simulink model "groundContactTestHarness"  (R2024a)
settings: configuration reference "standardSILConfiguraitonParams" (kept outside this file)
settings Model: Creator=jerem  LastModifiedBy=jerem
settings ConfigSetRef: SourceName=standardSILConfiguraitonParams  SourceLocation=Base Workspace

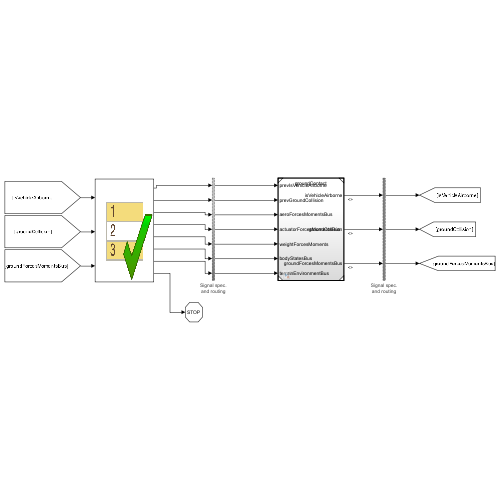
[thumbnail: Simulink's stored preview of the top-level diagram]
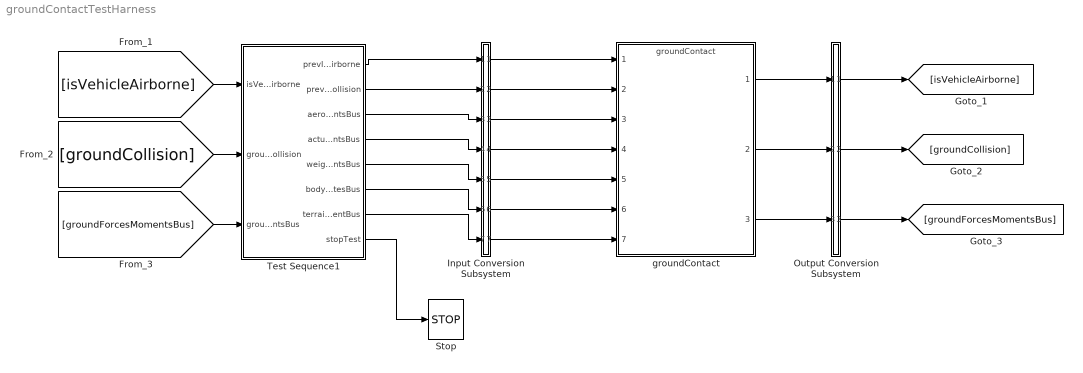
== system groundContactTestHarness ==
  Input Conversion Subsystem : Subsystem  Tag=__SLT_ICS__  Description=|
      | Signal spec.
      | and routing
      settings: AttributesFormatString=%<Description>
  Output Conversion Subsystem : Subsystem  Tag=__SLT_OCS__  Description=|
      | Signal spec.
      | and routing
      mask init:
      | ICDictionary = get_param(bdroot, 'DataDictionary');
      | if isempty(ICDictionary)
      |    ICScope = Simulink.data.BaseWorkspace;
      | else
      |    ICScope = Simulink.data.DataDictionary(ICDictionary);
      | end
      | 
      | IC3 = Simulink.Bus.createMATLABStruct('ComponentForcesMomentsBus', [], [1 1], ICScope);
      settings: AttributesFormatString=%<Description>
  Stop : Stop
  Test Sequence1 : Test Sequence  TreatAsAtomicUnit=on
  groundContact : ModelReference  ModelNameDialog=groundContact  SimulationMode=Normal  ModelReferenceVersion=1.95
  wires:
  Test Sequence1/1(prevIsVehicleAirborne) -> Input Conversion Subsystem/1(Inport_1)
  Test Sequence1/2(prevGroundCollision) -> Input Conversion Subsystem/2(Inport_2)
  Test Sequence1/3(aeroForcesMomentsBus) -> Input Conversion Subsystem/3(Inport_3)
  Test Sequence1/4(actuatorForcesMomentsBus) -> Input Conversion Subsystem/4(Inport_4)
  Test Sequence1/5(weightForcesMomentsBus) -> Input Conversion Subsystem/5(Inport_5)
  Test Sequence1/6(bodyStatesBus) -> Input Conversion Subsystem/6(Inport_6)
  Test Sequence1/7(terrainEnvironmentBus) -> Input Conversion Subsystem/7(Inport_7)
  [isVehicleAirborne] -> Test Sequence1/1(isVehicleAirborne)
  [groundCollision] -> Test Sequence1/2(groundCollision)
  [groundForcesMomentsBus] -> Test Sequence1/3(groundForcesMomentsBus)
  Output Conversion Subsystem/1(Outport_1) -> [isVehicleAirborne]
  Output Conversion Subsystem/2(Outport_2) -> [groundCollision]
  Output Conversion Subsystem/3(Outport_3) -> [groundForcesMomentsBus]
  Test Sequence1/8(stopTest) -> Stop/1
  groundContact/1 -> Output Conversion Subsystem/1(Inport_1)
  groundContact/2 -> Output Conversion Subsystem/2(Inport_2)
  groundContact/3 -> Output Conversion Subsystem/3(Inport_3)
  Input Conversion Subsystem/1(Outport_1) -> groundContact/1
  Input Conversion Subsystem/2(Outport_2) -> groundContact/2
  Input Conversion Subsystem/3(Outport_3) -> groundContact/3
  Input Conversion Subsystem/4(Outport_4) -> groundContact/4
  Input Conversion Subsystem/5(Outport_5) -> groundContact/5
  Input Conversion Subsystem/6(Outport_6) -> groundContact/6
  Input Conversion Subsystem/7(Outport_7) -> groundContact/7

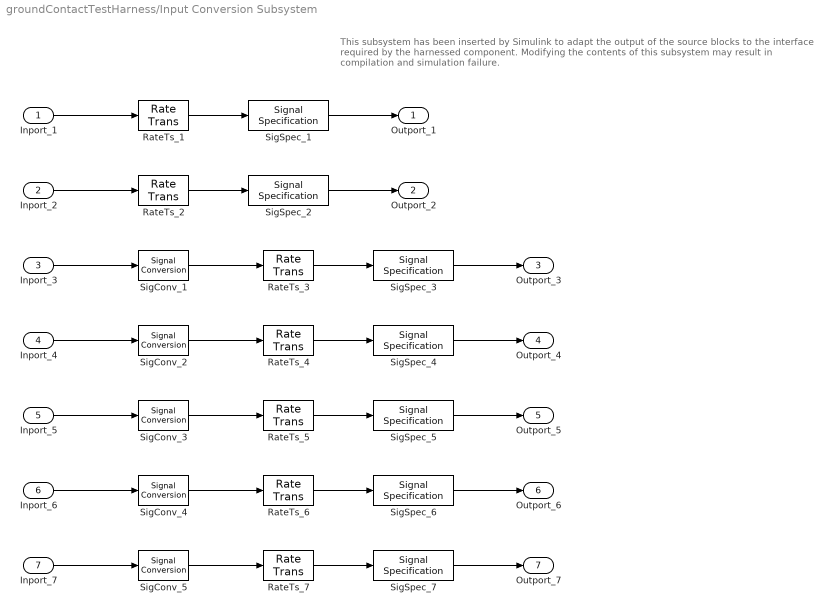
== system groundContactTestHarness/Input Conversion Subsystem ==
  note: This subsystem has been inserted by Simulink to adapt the output of the source blocks to the interface required by the harnessed component.
      |  Modifying the contents of this subsystem may result in compilation and simulation failure.
  Inport_1 : Inport
  Inport_2 : Inport  Port=2
  Inport_3 : Inport  Port=3
  Inport_4 : Inport  Port=4
  Inport_5 : Inport  Port=5
  Inport_6 : Inport  Port=6
  Inport_7 : Inport  Port=7
  RateTs_{1..7} (7 alike) : RateTransition  OutPortSampleTime=0.004
  SigConv_{1..5} (5 alike) : SignalConversion  ConversionOutput=Virtual bus  OverrideOpt=off
  SigSpec_1 : SignalSpecification  OutDataTypeStr=boolean  Dimensions=[1]  SampleTime=0.004
  SigSpec_2 : SignalSpecification  OutDataTypeStr=boolean  Dimensions=[1]  SampleTime=0.004
  SigSpec_3 : SignalSpecification  OutDataTypeStr=Bus: ComponentForcesMomentsBus  SampleTime=0.004
  SigSpec_4 : SignalSpecification  OutDataTypeStr=Bus: ComponentForcesMomentsBus  SampleTime=0.004
  SigSpec_5 : SignalSpecification  OutDataTypeStr=Bus: ComponentForcesMomentsBus  SampleTime=0.004
  SigSpec_6 : SignalSpecification  OutDataTypeStr=Bus: BodyStateBus  SampleTime=0.004
  SigSpec_7 : SignalSpecification  OutDataTypeStr=Bus: TerrainEnvironmentBus  SampleTime=0.004
  Outport_1 : Outport
  Outport_2 : Outport  Port=2
  Outport_3 : Outport  Port=3
  Outport_4 : Outport  Port=4
  Outport_5 : Outport  Port=5
  Outport_6 : Outport  Port=6
  Outport_7 : Outport  Port=7
  wires:
  SigSpec_1/1 -> Outport_1/1
  RateTs_1/1 -> SigSpec_1/1
  Inport_1/1 -> RateTs_1/1
  SigSpec_2/1 -> Outport_2/1
  RateTs_2/1 -> SigSpec_2/1
  Inport_2/1 -> RateTs_2/1
  SigSpec_3/1 -> Outport_3/1
  RateTs_3/1 -> SigSpec_3/1
  SigConv_1/1 -> RateTs_3/1
  Inport_3/1 -> SigConv_1/1
  SigSpec_4/1 -> Outport_4/1
  RateTs_4/1 -> SigSpec_4/1
  SigConv_2/1 -> RateTs_4/1
  Inport_4/1 -> SigConv_2/1
  SigSpec_5/1 -> Outport_5/1
  RateTs_5/1 -> SigSpec_5/1
  SigConv_3/1 -> RateTs_5/1
  Inport_5/1 -> SigConv_3/1
  SigSpec_6/1 -> Outport_6/1
  RateTs_6/1 -> SigSpec_6/1
  SigConv_4/1 -> RateTs_6/1
  Inport_6/1 -> SigConv_4/1
  SigSpec_7/1 -> Outport_7/1
  RateTs_7/1 -> SigSpec_7/1
  SigConv_5/1 -> RateTs_7/1
  Inport_7/1 -> SigConv_5/1

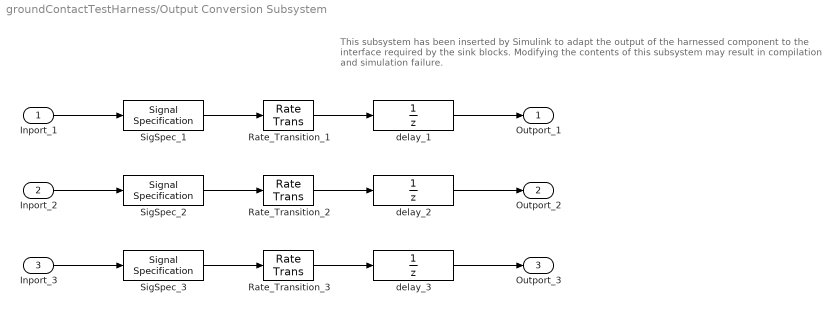
== system groundContactTestHarness/Output Conversion Subsystem ==
  note: This subsystem has been inserted by Simulink to adapt the output of the harnessed component to the interface required by the sink blocks.
      |  Modifying the contents of this subsystem may result in compilation and simulation failure.
  Inport_1 : Inport
  Inport_2 : Inport  Port=2
  Inport_3 : Inport  Port=3
  Rate_Transition_1 : RateTransition  OutPortSampleTimeOpt=Inherit
  Rate_Transition_2 : RateTransition  OutPortSampleTimeOpt=Inherit
  Rate_Transition_3 : RateTransition  OutPortSampleTimeOpt=Inherit
  SigSpec_1 : SignalSpecification  OutDataTypeStr=boolean  Dimensions=[1]  SampleTime=0.004
  SigSpec_2 : SignalSpecification  OutDataTypeStr=boolean  Dimensions=[1]  SampleTime=0.004
  SigSpec_3 : SignalSpecification  OutDataTypeStr=Bus: ComponentForcesMomentsBus  Dimensions=[1]  SampleTime=0.004
  delay_1 : UnitDelay  SampleTime=-1
  delay_2 : UnitDelay  SampleTime=-1
  delay_3 : UnitDelay  InitialCondition=IC3  SampleTime=-1
  Outport_1 : Outport
  Outport_2 : Outport  Port=2
  Outport_3 : Outport  Port=3
  wires:
  Inport_1/1 -> SigSpec_1/1
  SigSpec_1/1 -> Rate_Transition_1/1
  Rate_Transition_1/1 -> delay_1/1
  delay_1/1 -> Outport_1/1
  Inport_2/1 -> SigSpec_2/1
  SigSpec_2/1 -> Rate_Transition_2/1
  Rate_Transition_2/1 -> delay_2/1
  delay_2/1 -> Outport_2/1
  Inport_3/1 -> SigSpec_3/1
  SigSpec_3/1 -> Rate_Transition_3/1
  Rate_Transition_3/1 -> delay_3/1
  delay_3/1 -> Outport_3/1

== stateflow chart groundContactTestHarness/Test Sequence1 ==
  state Scenario_2
    state Initialize
      %% Initialize data outputs.
      stopTest = false;
      prevIsVehicleAirborne = false;
      prevGroundCollision = false;
      aeroForcesMomentsBus.forcesInBody_N = zeros(3,1);
      aeroForcesMomentsBus.momentsInBody_Nm = zeros(3,1);
      actuatorForcesMomentsBus.forcesInBody_N = zeros(3,1);
      actuatorForcesMomentsBus.momentsInBody_Nm = zeros(3,1);
      weightForcesMomentsBus.forcesInBody_N = zeros(3,1);
      weightForcesMomentsBus.momentsInBody_Nm = zeros(3,1);
      bodyStatesBus.aircraftVelInNED_mps = zeros(3,1);
      bodyStatesBus.aircraftPosInNED_m = zeros(3,1);
      bodyStatesBus.aircraftEulerAngles_rad = zeros(3,1);
      bodyStatesBus.aircraftVelInBody_mps = zeros(3,1);
      bodyStatesBus.aircraftAngVelInBody_radps = zeros(3,1);
      bodyStatesBus.aircraftAngAccelInBody_radps2 = zeros(3,1);
      bodyStatesBus.aircraftAccelInBody_mps2 = zeros(3,1);
      bodyStatesBus.DCM_be = eye(3,3);
      terrainEnvironmentBus.terrainHeightInNED_m = 0;
    state verifyInitialization
      verify(isVehicleAirborne == 0)
      verify(groundCollision == 0)
      verify(isClose(groundForcesMomentsBus.forcesInBody_N(1),0))
      verify(isClose(groundForcesMomentsBus.forcesInBody_N(2),0))
      verify(isClose(groundForcesMomentsBus.forcesInBody_N(3),0))
      verify(isClose(groundForcesMomentsBus.momentsInBody_Nm(1), 0))
      verify(isClose(groundForcesMomentsBus.momentsInBody_Nm(2), 0))
      verify(isClose(groundForcesMomentsBus.momentsInBody_Nm(3), 0))
    state stationaryOnAirstrip
      bodyStatesBus.DCM_be =  eye(3,3);
      % test some forces and moments
      aeroForcesMomentsBus.forcesInBody_N = [0; 0 ; 0]; % simulating moving on runway
      aeroForcesMomentsBus.momentsInBody_Nm = [0; 0; 0]; % Cm is naturally negative
      weightForcesMomentsBus.forcesInBody_N =[0; 0; 9298.6 * 9.81]; % weight of vehicle, must be positive (toward earth)
      weightForcesMomentsBus.momentsInBody_Nm = zeros(3,1);
    state verifyStationary
      verify(isVehicleAirborne == 0)
      verify(groundCollision == 0)
      verify(isClose(groundForcesMomentsBus.forcesInBody_N(1), 0))
      verify(isClose(groundForcesMomentsBus.forcesInBody_N(2), 0))
      verify(isClose(groundForcesMomentsBus.forcesInBody_N(3), -9298.6 * 9.81 ))
      verify(isClose(weightForcesMomentsBus.momentsInBody_Nm(1), 0))
      verify(isClose(weightForcesMomentsBus.momentsInBody_Nm(2), 0))
      verify(isClose(weightForcesMomentsBus.momentsInBody_Nm(3), 0))
    state fastTaxi
      bodyStatesBus.DCM_be =  eye(3,3);
      % test some forces and moments
      aeroForcesMomentsBus.forcesInBody_N = [-400; 0 ; -20000]; % simulating moving on runway
      aeroForcesMomentsBus.momentsInBody_Nm = [0; -20; 0]; % Cm is naturally negative
      weightForcesMomentsBus.forcesInBody_N =[0; 0; 9298.6 * 9.81]; % weight of vehicle
      weightForcesMomentsBus.momentsInBody_Nm = zeros(3,1);
    state verifyFastTaxi
      verify(isVehicleAirborne == 0)
      verify(groundCollision == 0)
      verify(isClose(groundForcesMomentsBus.forcesInBody_N(1), 0)) %This should never be non-zero because ground forces only impact Z-axis
      verify(isClose(groundForcesMomentsBus.forcesInBody_N(2), 0))
      verify(isClose(groundForcesMomentsBus.forcesInBody_N(3), -9298.6 * 9.81 + 20000 ))
      verify(isClose(groundForcesMomentsBus.momentsInBody_Nm(1),0))
      verify(isClose(groundForcesMomentsBus.momentsInBody_Nm(2),0))
      verify(isClose(groundForcesMomentsBus.momentsInBody_Nm(3),0))
      verify(isClose(weightForcesMomentsBus.momentsInBody_Nm(1), 0))
      verify(isClose(weightForcesMomentsBus.momentsInBody_Nm(2), 0))
      verify(isClose(weightForcesMomentsBus.momentsInBody_Nm(3), 0))
    state rotate
      aeroForcesMomentsBus.momentsInBody_Nm = [0; 20; 0]; % Emulate a positive pitch moment
    state verifyRotate
      verify(isVehicleAirborne == 0)
      verify(groundCollision == 0)
      verify(isClose(groundForcesMomentsBus.forcesInBody_N(1), 0)) %This should never be non-zero because ground forces only impact Z-axis
      verify(isClose(groundForcesMomentsBus.forcesInBody_N(2), 0))
      verify(isClose(groundForcesMomentsBus.forcesInBody_N(3), -9298.6 * 9.81 + 20000 ))
      verify(isClose(groundForcesMomentsBus.momentsInBody_Nm(1),0))
      verify(isClose(groundForcesMomentsBus.momentsInBody_Nm(2),0)) % ground should allow vehicle to pitch up
      verify(isClose(groundForcesMomentsBus.momentsInBody_Nm(3),0))
      verify(isClose(weightForcesMomentsBus.momentsInBody_Nm(1), 0))
      verify(isClose(weightForcesMomentsBus.momentsInBody_Nm(2), 0))
      verify(isClose(weightForcesMomentsBus.momentsInBody_Nm(3), 0))
    state takeoff
      % test some forces and moments
      aeroForcesMomentsBus.forcesInBody_N = [-400; 0 ; -100000]; % simulating moving on runway
      bodyStatesBus.aircraftPosInNED_m(3) = -1;
    state verifyTakeoff
      verify(isVehicleAirborne == 1)
      verify(groundCollision == 0)
      verify(isClose(groundForcesMomentsBus.forcesInBody_N(1), 0))
      verify(isClose(groundForcesMomentsBus.forcesInBody_N(2), 0))
      verify(isClose(groundForcesMomentsBus.forcesInBody_N(3), 0))
      verify(isClose(groundForcesMomentsBus.momentsInBody_Nm(1),0))
      verify(isClose(groundForcesMomentsBus.momentsInBody_Nm(2),0))
      verify(isClose(groundForcesMomentsBus.momentsInBody_Nm(3),0))
      verify(isClose(weightForcesMomentsBus.momentsInBody_Nm(1), 0))
      verify(isClose(weightForcesMomentsBus.momentsInBody_Nm(2), 0))
      verify(isClose(weightForcesMomentsBus.momentsInBody_Nm(3), 0))
    state EndTest
      stopTest = true;
    (default) -> Initialize
    Initialize -> verifyInitialization : [
        | after(0.5,sec)
        | ]
    verifyInitialization -> stationaryOnAirstrip : [
        | true
        | ]
    stationaryOnAirstrip -> verifyStationary : [
        | after(0.5,sec)
        | ]
    verifyStationary -> fastTaxi : [
        | after(1,tick)
        | ]
    fastTaxi -> verifyFastTaxi : [
        | after(1,sec)
        | ]
    verifyFastTaxi -> rotate : [
        | after(1,tick)
        | ]
    rotate -> verifyRotate : [
        | after(1,tick)
        | ]
    verifyRotate -> takeoff : [
        | after(1,tick)
        | ]
    takeoff -> verifyTakeoff : [
        | after(1,tick)
        | ]
    verifyTakeoff -> EndTest : [
        | after(1,tick)
        | ]
  (default) -> Scenario_2 : {assert(Active_Scenario_Index == 1,'The value of Scenario Parameter ''Active_Scenario_Index'' is not valid. Use the index of the scenario to specify it.')}
  data: isVehicleAirborne input boolean size=[1]; groundCollision input boolean size=[1]; groundForcesMomentsBus input Bus: ComponentForcesMomentsBus size=[1]; prevIsVehicleAirborne output boolean size=[1]; prevGroundCollision output boolean size=[1]; aeroForcesMomentsBus output Bus: ComponentForcesMomentsBus size=[1]; actuatorForcesMomentsBus output Bus: ComponentForcesMomentsBus size=[1]; weightForcesMomentsBus output Bus: ComponentForcesMomentsBus size=[1]; bodyStatesBus output Bus: BodyStateBus size=[1]; terrainEnvironmentBus output Bus: TerrainEnvironmentBus size=[1]; Active_Scenario_Index parameter =1; stopTest output
